simulink model "RELOrigin"  (R2022a)
settings: configuration reference "ChildModel" (kept outside this file)
libraries: simulink x4
(part 2 of 2)

== stateflow chart RELOrigin/REL/FRCenDoorRat ==
  state Initial
    en:
    SO_b_DoorRatRelaseReq=0;
    SO_DLKUnlockReq=0;
  state TRIGGER
    state DOOR_LOCK
      state REQ_UNLOCK
        en:
        SO_DLKUnlockReq=1;
      state SUCESS_UNLOCK
      state FAIL_UNLOCK
      (default) -> REQ_UNLOCK
      REQ_UNLOCK -> SUCESS_UNLOCK [order 1] : [SI_e_DoorLockSts==1]
      REQ_UNLOCK -> FAIL_UNLOCK [order 2] : [after(100,tick)&&...
          | SI_e_DoorLockSts==0]
    state RELEASE
      en:
      SO_b_DoorRatRelaseReq=1;
    state DOOR_UNLOCK
    (default) -> DOOR_LOCK [order 1] : [SI_e_DoorLockSts==0]
    DOOR_LOCK -> RELEASE : [SI_e_DoorLockSts==1&&...
        | SI_e_DoorRatSts!=3]
    DOOR_UNLOCK -> RELEASE : [SI_e_DoorLockSts==1&&...
        | SI_e_DoorRatSts!=3]
    (default) -> DOOR_UNLOCK [order 2]
  (default) -> Initial
  Initial -> TRIGGER : [!SI_b_OFF&&...
      | SI_e_DoorRatSts!=3&&...
      | ((SI_e_EspVehSpd<=0&&SI_b_EspVehSpdVld==0)||...
      | SI_e_VcuGearPosn==1)&&...
      | (hasChangedTo(SI_b_CdcDoorButtonSts,1)||...
      | hasChangedTo(SI_b_Cdc4DoorOpenButtonSts,1))]
  TRIGGER -> Initial : [hasChangedFrom(SI_e_VcuGearPosn,1)||...
      | (SI_e_EspVehSpd>=5&&SI_b_EspVehSpdVld==0)||...
      | (after(105,tick)&&SI_e_DoorLockSts==0)]
  RELEASE -> (junction 82) : [after(5,tick)]
  (junction 82) -> Initial
  data: SI_b_OFF input boolean; SO_b_DoorRatRelaseReq output boolean; SI_e_DoorLockSts input uint8; SI_e_EspVehSpd input uint8; SI_b_EspVehSpdVld input boolean; SI_e_DoorRatSts input uint8; SO_DLKUnlockReq output boolean; SI_e_VcuGearPosn input uint8; SI_b_CdcDoorButtonSts input boolean; SI_b_Cdc4DoorOpenButtonSts input boolean

== stateflow chart RELOrigin/REL/RLElecDoorRat ==
  state Initial
    en:
    SO_b_DoorRatRelaseReq=0;
  state RELEASE
    en:
    SO_b_DoorRatRelaseReq=1;
  (default) -> Initial
  Initial -> RELEASE : [!SI_b_OFF&&...
      | SI_e_DoorLockSts==1&&...
      | SI_e_DoorRatSts!=3&&...
      | ((SI_e_EspVehSpd<=0&&SI_b_EspVehSpdVld==0)||...
      | SI_e_VcuGearPosn==1)&&...
      | ((SI_e_BDCDoorHndSts==1&&hasChangedTo(SI_b_DoorHandleSW,1))||...
      | (SI_e_VcuGearPosn==1&&hasChangedTo(SI_e_BTDoorOpenReq,5))||...
      | (SI_e_VcuGearPosn==1&&hasChangedTo(SI_e_BTDoorOpenReq,9)))]
  RELEASE -> Initial : [after(5,tick)]
  data: SI_b_OFF input boolean; SO_b_DoorRatRelaseReq output boolean; SI_e_DoorLockSts input uint8; SI_e_EspVehSpd input uint8; SI_b_EspVehSpdVld input boolean; SI_e_DoorRatSts input uint8; SI_e_VcuGearPosn input uint8; SI_e_BDCDoorHndSts input uint8; SI_b_DoorHandleSW input boolean; SI_e_BTDoorOpenReq input uint8

== stateflow chart RELOrigin/REL/RLCenDoorRat ==
  state Initial
    en:
    SO_b_DoorRatRelaseReq=0;
    SO_DLKUnlockReq=0;
  state TRIGGER
    state DOOR_LOCK
      state REQ_UNLOCK
        en:
        SO_DLKUnlockReq=1;
      state SUCESS_UNLOCK
      state FAIL_UNLOCK
      (default) -> REQ_UNLOCK
      REQ_UNLOCK -> SUCESS_UNLOCK [order 1] : [SI_e_DoorLockSts==1]
      REQ_UNLOCK -> FAIL_UNLOCK [order 2] : [after(100,tick)&&...
          | SI_e_DoorLockSts==0]
    state RELEASE
      en:
      SO_b_DoorRatRelaseReq=1;
    state DOOR_UNLOCK
    (default) -> DOOR_LOCK [order 1] : [SI_e_DoorLockSts==0]
    DOOR_LOCK -> RELEASE : [SI_e_DoorLockSts==1&&...
        | SI_e_DoorRatSts!=3]
    DOOR_UNLOCK -> RELEASE : [SI_e_DoorLockSts==1&&...
        | SI_e_DoorRatSts!=3]
    (default) -> DOOR_UNLOCK [order 2]
  (default) -> Initial
  Initial -> TRIGGER : [!SI_b_OFF&&...
      | SI_e_DoorRatSts!=3&&...
      | ((SI_e_EspVehSpd<=0&&SI_b_EspVehSpdVld==0)||...
      | SI_e_VcuGearPosn==1)&&...
      | (hasChangedTo(SI_b_CdcDoorButtonSts,1)||...
      | hasChangedTo(SI_b_Cdc4DoorOpenButtonSts,1))]
  TRIGGER -> Initial : [hasChangedFrom(SI_e_VcuGearPosn,1)||...
      | (SI_e_EspVehSpd>=5&&SI_b_EspVehSpdVld==0)||...
      | (after(105,tick)&&SI_e_DoorLockSts==0)]
  RELEASE -> (junction 82) : [after(5,tick)]
  (junction 82) -> Initial
  data: SI_b_OFF input boolean; SO_b_DoorRatRelaseReq output boolean; SI_e_DoorLockSts input uint8; SI_e_EspVehSpd input uint8; SI_b_EspVehSpdVld input boolean; SI_e_DoorRatSts input uint8; SO_DLKUnlockReq output boolean; SI_e_VcuGearPosn input uint8; SI_b_CdcDoorButtonSts input boolean; SI_b_Cdc4DoorOpenButtonSts input boolean

== stateflow chart RELOrigin/REL/RRElecDoorRat ==
  state Initial
    en:
    SO_b_DoorRatRelaseReq=0;
  state RELEASE
    en:
    SO_b_DoorRatRelaseReq=1;
  (default) -> Initial
  Initial -> RELEASE : [!SI_b_OFF&&...
      | SI_e_DoorLockSts==1&&...
      | SI_e_DoorRatSts!=3&&...
      | ((SI_e_EspVehSpd<=0&&SI_b_EspVehSpdVld==0)||...
      | SI_e_VcuGearPosn==1)&&...
      | ((SI_e_BDCDoorHndSts==1&&hasChangedTo(SI_b_DoorHandleSW,1))||...
      | (SI_e_VcuGearPosn==1&&hasChangedTo(SI_e_BTDoorOpenReq,7))||...
      | (SI_e_VcuGearPosn==1&&hasChangedTo(SI_e_BTDoorOpenReq,9)))]
  RELEASE -> Initial : [after(5,tick)]
  data: SI_b_OFF input boolean; SO_b_DoorRatRelaseReq output boolean; SI_e_DoorLockSts input uint8; SI_e_EspVehSpd input uint8; SI_b_EspVehSpdVld input boolean; SI_e_DoorRatSts input uint8; SI_e_VcuGearPosn input uint8; SI_e_BDCDoorHndSts input uint8; SI_b_DoorHandleSW input boolean; SI_e_BTDoorOpenReq input uint8

== stateflow chart RELOrigin/REL/RRCenDoorRat ==
  state Initial
    en:
    SO_b_DoorRatRelaseReq=0;
    SO_DLKUnlockReq=0;
  state TRIGGER
    state DOOR_LOCK
      state REQ_UNLOCK
        en:
        SO_DLKUnlockReq=1;
      state SUCESS_UNLOCK
      state FAIL_UNLOCK
      (default) -> REQ_UNLOCK
      REQ_UNLOCK -> SUCESS_UNLOCK [order 1] : [SI_e_DoorLockSts==1]
      REQ_UNLOCK -> FAIL_UNLOCK [order 2] : [after(100,tick)&&...
          | SI_e_DoorLockSts==0]
    state RELEASE
      en:
      SO_b_DoorRatRelaseReq=1;
    state DOOR_UNLOCK
    (default) -> DOOR_LOCK [order 1] : [SI_e_DoorLockSts==0]
    DOOR_LOCK -> RELEASE : [SI_e_DoorLockSts==1&&...
        | SI_e_DoorRatSts!=3]
    DOOR_UNLOCK -> RELEASE : [SI_e_DoorLockSts==1&&...
        | SI_e_DoorRatSts!=3]
    (default) -> DOOR_UNLOCK [order 2]
  (default) -> Initial
  Initial -> TRIGGER : [!SI_b_OFF&&...
      | SI_e_DoorRatSts!=3&&...
      | ((SI_e_EspVehSpd<=0&&SI_b_EspVehSpdVld==0)||...
      | SI_e_VcuGearPosn==1)&&...
      | (hasChangedTo(SI_b_CdcDoorButtonSts,1)||...
      | hasChangedTo(SI_b_Cdc4DoorOpenButtonSts,1))]
  TRIGGER -> Initial : [hasChangedFrom(SI_e_VcuGearPosn,1)||...
      | (SI_e_EspVehSpd>=5&&SI_b_EspVehSpdVld==0)||...
      | (after(105,tick)&&SI_e_DoorLockSts==0)]
  RELEASE -> (junction 82) : [after(5,tick)]
  (junction 82) -> Initial
  data: SI_b_OFF input boolean; SO_b_DoorRatRelaseReq output boolean; SI_e_DoorLockSts input uint8; SI_e_EspVehSpd input uint8; SI_b_EspVehSpdVld input boolean; SI_e_DoorRatSts input uint8; SO_DLKUnlockReq output boolean; SI_e_VcuGearPosn input uint8; SI_b_CdcDoorButtonSts input boolean; SI_b_Cdc4DoorOpenButtonSts input boolean

== stateflow chart RELOrigin/REL/FLDoorReleaseDriver ==
  state STARTUP_SETTING
    en:
    SO_b_MotorA=0;
    SO_b_MotorB=1;
    SO_e_MotorMode=2;
  state NORMAL
    state ELECTRIC_DOOR
      state MAIN_PROGRESS [parallel]
        settings: executionOrder=1
        state RELEASE
          en:
          SL_e_CheckCycle=0;
          state STEP2_OPEN
            state IDLE
              en:
              SO_b_MotorA=0;
              SO_b_MotorB=0;
              SO_e_MotorMode=0;
            state WAITING
            state ERROR
              en:
              SO_b_Error=1;
            state LAST_CHECK
            state ICE_BREAK
            state ERROR1
              en:
              SO_b_Error=1;
            (default) -> NORMAL.ELECTRIC_DOOR.MAIN_PROGRESS.RELEASE.STEP2_OPEN.IDLE
            NORMAL.ELECTRIC_DOOR.MAIN_PROGRESS.RELEASE.STEP2_OPEN.IDLE -> NORMAL.ELECTRIC_DOOR.MAIN_PROGRESS.RELEASE.STEP2_OPEN.WAITING [order 1] : [SI_b_DoorOpenSts==1]
            NORMAL.ELECTRIC_DOOR.MAIN_PROGRESS.RELEASE.STEP2_OPEN.WAITING -> (junction 227) : [after(5,tick)]
            (junction 227) -> (junction 226)
            NORMAL.ELECTRIC_DOOR.MAIN_PROGRESS.RELEASE.STEP2_OPEN.IDLE -> (junction 226) [order 2] : [before(270,tick)&&...
                | hasChangedTo(SI_b_DoorOpenSts,1)]
            (junction 226) -> (junction 219)
            NORMAL.ELECTRIC_DOOR.MAIN_PROGRESS.RELEASE.STEP2_OPEN.IDLE -> NORMAL.ELECTRIC_DOOR.MAIN_PROGRESS.RELEASE.STEP2_OPEN.LAST_CHECK [order 3] : [after(300,tick)&&...
                | SI_b_DoorOpenSts==0]
            ERROR -> (junction 219) : [after(5,tick)]
            NORMAL.ELECTRIC_DOOR.MAIN_PROGRESS.RELEASE.STEP2_OPEN.LAST_CHECK -> ERROR [order 1] : [SI_b_DCUCinchHomeSwt!=1]
            (junction 219) -> (junction 210)
            NORMAL.ELECTRIC_DOOR.MAIN_PROGRESS.RELEASE.STEP2_OPEN.LAST_CHECK -> ICE_BREAK [order 2] : [SI_b_DCUCinchHomeSwt==1]
            ICE_BREAK -> ERROR1 [order 2] : [after(600,tick)&&...
                | SI_b_DCUCinchHomeSwt==1]
            ERROR1 -> (junction 210) : [after(5,tick)]
            (junction 210) -> (junction 225)
            ICE_BREAK -> (junction 225) [order 1] : [before(600,tick)&&...
                | hasChangedTo(SI_b_DCUCinchHomeSwt,0)]
          state INITIAL
            en:
            SO_b_MotorA=1;
            SO_b_MotorB=0;
            SO_e_MotorMode=1;
            //MotorA=Release Side
          state CHECKING
            en:
            SO_b_MotorA=0;
            SO_b_MotorB=0;
            SO_e_MotorMode=0;
            SL_e_CheckCycle++;
          state RESET
            en:
            SO_b_MotorA=0;
            SO_b_MotorB=1;
            SO_e_MotorMode=2;
          (default) -> NORMAL.ELECTRIC_DOOR.MAIN_PROGRESS.RELEASE.INITIAL
          NORMAL.ELECTRIC_DOOR.MAIN_PROGRESS.RELEASE.INITIAL -> NORMAL.ELECTRIC_DOOR.MAIN_PROGRESS.RELEASE.CHECKING : [after(30,tick)]
          NORMAL.ELECTRIC_DOOR.MAIN_PROGRESS.RELEASE.CHECKING -> NORMAL.ELECTRIC_DOOR.MAIN_PROGRESS.RELEASE.INITIAL [order 2] : [after(5,tick)&&...
              | SI_b_DoorAjarSts!=1&&...
              | SL_e_CheckCycle<2]
          NORMAL.ELECTRIC_DOOR.MAIN_PROGRESS.RELEASE.CHECKING -> NORMAL.ELECTRIC_DOOR.MAIN_PROGRESS.RELEASE.STEP2_OPEN [order 1] : [after(5,tick)&&...
              | SI_b_DoorAjarSts==1]
          NORMAL.ELECTRIC_DOOR.MAIN_PROGRESS.RELEASE.CHECKING -> NORMAL.ELECTRIC_DOOR.MAIN_PROGRESS.RELEASE.RESET [order 3] : [after(5,tick)&&...
              | SI_b_DoorAjarSts!=1&&...
              | SL_e_CheckCycle>=2]
          (junction 225) -> NORMAL.ELECTRIC_DOOR.MAIN_PROGRESS.RELEASE.RESET
        state IDLE
          en:
          SO_b_MotorA=0;
          SO_b_MotorB=0;
          SO_e_MotorMode=0;
          SO_b_Error=0;
        (default) -> NORMAL.ELECTRIC_DOOR.MAIN_PROGRESS.IDLE
        NORMAL.ELECTRIC_DOOR.MAIN_PROGRESS.IDLE -> NORMAL.ELECTRIC_DOOR.MAIN_PROGRESS.RELEASE : [hasChangedTO(SI_b_TriggerRelease,1)]
        NORMAL.ELECTRIC_DOOR.MAIN_PROGRESS.RELEASE.RESET -> NORMAL.ELECTRIC_DOOR.MAIN_PROGRESS.IDLE : [after(30,tick)]
    state NON_ELECTRIC_DOOR
      state MAIN_PROGRESS [parallel]
        settings: executionOrder=1
        state RELEASE
          en:
          SL_e_CheckCycle=0;
          state INITIAL
            en:
            SO_b_MotorA=1;
            SO_b_MotorB=0;
            SO_e_MotorMode=1;
            //MotorA=Release Side
          state CHECKING
            en:
            SO_b_MotorA=0;
            SO_b_MotorB=0;
            SO_e_MotorMode=0;
            SL_e_CheckCycle++;
          state STEP2_OPEN
            state IDLE
              en:
              SO_b_MotorA=0;
              SO_b_MotorB=0;
              SO_e_MotorMode=0;
            state WAITING
            state LAST_CHECK
            (default) -> NORMAL.NON_ELECTRIC_DOOR.MAIN_PROGRESS.RELEASE.STEP2_OPEN.IDLE
            NORMAL.NON_ELECTRIC_DOOR.MAIN_PROGRESS.RELEASE.STEP2_OPEN.WAITING -> (junction 251) : [after(5,tick)]
            NORMAL.NON_ELECTRIC_DOOR.MAIN_PROGRESS.RELEASE.STEP2_OPEN.IDLE -> NORMAL.NON_ELECTRIC_DOOR.MAIN_PROGRESS.RELEASE.STEP2_OPEN.WAITING [order 1] : [SI_b_DoorOpenSts==1]
            (junction 251) -> (junction 250)
            NORMAL.NON_ELECTRIC_DOOR.MAIN_PROGRESS.RELEASE.STEP2_OPEN.IDLE -> (junction 250) [order 2] : [before(270,tick)&&...
                | hasChangedTo(SI_b_DoorOpenSts,1)]
            (junction 250) -> (junction 242)
            NORMAL.NON_ELECTRIC_DOOR.MAIN_PROGRESS.RELEASE.STEP2_OPEN.IDLE -> NORMAL.NON_ELECTRIC_DOOR.MAIN_PROGRESS.RELEASE.STEP2_OPEN.LAST_CHECK [order 3] : [after(300,tick)&&...
                | SI_b_DoorOpenSts==0]
            NORMAL.NON_ELECTRIC_DOOR.MAIN_PROGRESS.RELEASE.STEP2_OPEN.LAST_CHECK -> (junction 242)
          state RESET
            en:
            SO_b_MotorA=0;
            SO_b_MotorB=1;
            SO_e_MotorMode=2;
          (default) -> NORMAL.NON_ELECTRIC_DOOR.MAIN_PROGRESS.RELEASE.INITIAL
          NORMAL.NON_ELECTRIC_DOOR.MAIN_PROGRESS.RELEASE.INITIAL -> NORMAL.NON_ELECTRIC_DOOR.MAIN_PROGRESS.RELEASE.CHECKING : [after(30,tick)]
          NORMAL.NON_ELECTRIC_DOOR.MAIN_PROGRESS.RELEASE.CHECKING -> NORMAL.NON_ELECTRIC_DOOR.MAIN_PROGRESS.RELEASE.STEP2_OPEN [order 1] : [after(5,tick)&&...
              | SI_b_DoorAjarSts==1]
          NORMAL.NON_ELECTRIC_DOOR.MAIN_PROGRESS.RELEASE.CHECKING -> NORMAL.NON_ELECTRIC_DOOR.MAIN_PROGRESS.RELEASE.INITIAL [order 2] : [after(5,tick)&&...
              | SI_b_DoorAjarSts!=1&&...
              | SL_e_CheckCycle<2]
          NORMAL.NON_ELECTRIC_DOOR.MAIN_PROGRESS.RELEASE.CHECKING -> NORMAL.NON_ELECTRIC_DOOR.MAIN_PROGRESS.RELEASE.RESET [order 3] : [after(5,tick)&&...
              | SI_b_DoorAjarSts!=1&&...
              | SL_e_CheckCycle>=2]
          (junction 242) -> NORMAL.NON_ELECTRIC_DOOR.MAIN_PROGRESS.RELEASE.RESET
        state IDLE
          en:
          SO_b_MotorA=0;
          SO_b_MotorB=0;
          SO_e_MotorMode=0;
        (default) -> NORMAL.NON_ELECTRIC_DOOR.MAIN_PROGRESS.IDLE
        NORMAL.NON_ELECTRIC_DOOR.MAIN_PROGRESS.IDLE -> NORMAL.NON_ELECTRIC_DOOR.MAIN_PROGRESS.RELEASE : [hasChangedTO(SI_b_TriggerRelease,1)]
        NORMAL.NON_ELECTRIC_DOOR.MAIN_PROGRESS.RELEASE.RESET -> NORMAL.NON_ELECTRIC_DOOR.MAIN_PROGRESS.IDLE : [after(30,tick)]
    (default) -> ELECTRIC_DOOR [order 1] : [SI_b_ElectricDoorCfg]
    (default) -> NON_ELECTRIC_DOOR [order 2]
  (default) -> STARTUP_SETTING
  STARTUP_SETTING -> NORMAL : [after(30,tick)]
  data: SO_b_MotorA output boolean; SI_b_TriggerRelease input boolean; SI_b_DoorOpenSts input boolean; SO_b_MotorB output boolean; SO_e_MotorMode output uint8; SI_b_DCUCinchHomeSwt input boolean; SO_b_Error output boolean; SI_b_ElectricDoorCfg input boolean; SI_b_DoorAjarSts input boolean

== stateflow chart RELOrigin/REL/FRDoorReleaseDriver ==
  state STARTUP_SETTING
    en:
    SO_b_MotorA=0;
    SO_b_MotorB=1;
    SO_e_MotorMode=2;
  state NORMAL
    state ELECTRIC_DOOR
      state MAIN_PROGRESS [parallel]
        settings: executionOrder=1
        state RELEASE
          en:
          SL_e_CheckCycle=0;
          state STEP2_OPEN
            state IDLE
              en:
              SO_b_MotorA=0;
              SO_b_MotorB=0;
              SO_e_MotorMode=0;
            state WAITING
            state ERROR
              en:
              SO_b_Error=1;
            state LAST_CHECK
            state ICE_BREAK
            state ERROR1
              en:
              SO_b_Error=1;
            (default) -> NORMAL.ELECTRIC_DOOR.MAIN_PROGRESS.RELEASE.STEP2_OPEN.IDLE
            NORMAL.ELECTRIC_DOOR.MAIN_PROGRESS.RELEASE.STEP2_OPEN.IDLE -> NORMAL.ELECTRIC_DOOR.MAIN_PROGRESS.RELEASE.STEP2_OPEN.WAITING [order 1] : [SI_b_DoorOpenSts==1]
            NORMAL.ELECTRIC_DOOR.MAIN_PROGRESS.RELEASE.STEP2_OPEN.WAITING -> (junction 227) : [after(5,tick)]
            (junction 227) -> (junction 226)
            NORMAL.ELECTRIC_DOOR.MAIN_PROGRESS.RELEASE.STEP2_OPEN.IDLE -> (junction 226) [order 2] : [before(270,tick)&&...
                | hasChangedTo(SI_b_DoorOpenSts,1)]
            (junction 226) -> (junction 219)
            NORMAL.ELECTRIC_DOOR.MAIN_PROGRESS.RELEASE.STEP2_OPEN.IDLE -> NORMAL.ELECTRIC_DOOR.MAIN_PROGRESS.RELEASE.STEP2_OPEN.LAST_CHECK [order 3] : [after(300,tick)&&...
                | SI_b_DoorOpenSts==0]
            ERROR -> (junction 219) : [after(5,tick)]
            NORMAL.ELECTRIC_DOOR.MAIN_PROGRESS.RELEASE.STEP2_OPEN.LAST_CHECK -> ERROR [order 1] : [SI_b_DCUCinchHomeSwt!=1]
            (junction 219) -> (junction 210)
            NORMAL.ELECTRIC_DOOR.MAIN_PROGRESS.RELEASE.STEP2_OPEN.LAST_CHECK -> ICE_BREAK [order 2] : [SI_b_DCUCinchHomeSwt==1]
            ICE_BREAK -> ERROR1 [order 2] : [after(600,tick)&&...
                | SI_b_DCUCinchHomeSwt==1]
            ERROR1 -> (junction 210) : [after(5,tick)]
            (junction 210) -> (junction 225)
            ICE_BREAK -> (junction 225) [order 1] : [before(600,tick)&&...
                | hasChangedTo(SI_b_DCUCinchHomeSwt,0)]
          state INITIAL
            en:
            SO_b_MotorA=1;
            SO_b_MotorB=0;
            SO_e_MotorMode=1;
            //MotorA=Release Side
          state CHECKING
            en:
            SO_b_MotorA=0;
            SO_b_MotorB=0;
            SO_e_MotorMode=0;
            SL_e_CheckCycle++;
          state RESET
            en:
            SO_b_MotorA=0;
            SO_b_MotorB=1;
            SO_e_MotorMode=2;
          (default) -> NORMAL.ELECTRIC_DOOR.MAIN_PROGRESS.RELEASE.INITIAL
          NORMAL.ELECTRIC_DOOR.MAIN_PROGRESS.RELEASE.INITIAL -> NORMAL.ELECTRIC_DOOR.MAIN_PROGRESS.RELEASE.CHECKING : [after(30,tick)]
          NORMAL.ELECTRIC_DOOR.MAIN_PROGRESS.RELEASE.CHECKING -> NORMAL.ELECTRIC_DOOR.MAIN_PROGRESS.RELEASE.INITIAL [order 2] : [after(5,tick)&&...
              | SI_b_DoorAjarSts!=1&&...
              | SL_e_CheckCycle<2]
          NORMAL.ELECTRIC_DOOR.MAIN_PROGRESS.RELEASE.CHECKING -> NORMAL.ELECTRIC_DOOR.MAIN_PROGRESS.RELEASE.STEP2_OPEN [order 1] : [after(5,tick)&&...
              | SI_b_DoorAjarSts==1]
          NORMAL.ELECTRIC_DOOR.MAIN_PROGRESS.RELEASE.CHECKING -> NORMAL.ELECTRIC_DOOR.MAIN_PROGRESS.RELEASE.RESET [order 3] : [after(5,tick)&&...
              | SI_b_DoorAjarSts!=1&&...
              | SL_e_CheckCycle>=2]
          (junction 225) -> NORMAL.ELECTRIC_DOOR.MAIN_PROGRESS.RELEASE.RESET
        state IDLE
          en:
          SO_b_MotorA=0;
          SO_b_MotorB=0;
          SO_e_MotorMode=0;
          SO_b_Error=0;
        (default) -> NORMAL.ELECTRIC_DOOR.MAIN_PROGRESS.IDLE
        NORMAL.ELECTRIC_DOOR.MAIN_PROGRESS.IDLE -> NORMAL.ELECTRIC_DOOR.MAIN_PROGRESS.RELEASE : [hasChangedTO(SI_b_TriggerRelease,1)]
        NORMAL.ELECTRIC_DOOR.MAIN_PROGRESS.RELEASE.RESET -> NORMAL.ELECTRIC_DOOR.MAIN_PROGRESS.IDLE : [after(30,tick)]
    state NON_ELECTRIC_DOOR
      state MAIN_PROGRESS [parallel]
        settings: executionOrder=1
        state RELEASE
          en:
          SL_e_CheckCycle=0;
          state INITIAL
            en:
            SO_b_MotorA=1;
            SO_b_MotorB=0;
            SO_e_MotorMode=1;
            //MotorA=Release Side
          state CHECKING
            en:
            SO_b_MotorA=0;
            SO_b_MotorB=0;
            SO_e_MotorMode=0;
            SL_e_CheckCycle++;
          state STEP2_OPEN
            state IDLE
              en:
              SO_b_MotorA=0;
              SO_b_MotorB=0;
              SO_e_MotorMode=0;
            state WAITING
            state LAST_CHECK
            (default) -> NORMAL.NON_ELECTRIC_DOOR.MAIN_PROGRESS.RELEASE.STEP2_OPEN.IDLE
            NORMAL.NON_ELECTRIC_DOOR.MAIN_PROGRESS.RELEASE.STEP2_OPEN.WAITING -> (junction 251) : [after(5,tick)]
            NORMAL.NON_ELECTRIC_DOOR.MAIN_PROGRESS.RELEASE.STEP2_OPEN.IDLE -> NORMAL.NON_ELECTRIC_DOOR.MAIN_PROGRESS.RELEASE.STEP2_OPEN.WAITING [order 1] : [SI_b_DoorOpenSts==1]
            (junction 251) -> (junction 250)
            NORMAL.NON_ELECTRIC_DOOR.MAIN_PROGRESS.RELEASE.STEP2_OPEN.IDLE -> (junction 250) [order 2] : [before(270,tick)&&...
                | hasChangedTo(SI_b_DoorOpenSts,1)]
            (junction 250) -> (junction 242)
            NORMAL.NON_ELECTRIC_DOOR.MAIN_PROGRESS.RELEASE.STEP2_OPEN.IDLE -> NORMAL.NON_ELECTRIC_DOOR.MAIN_PROGRESS.RELEASE.STEP2_OPEN.LAST_CHECK [order 3] : [after(300,tick)&&...
                | SI_b_DoorOpenSts==0]
            NORMAL.NON_ELECTRIC_DOOR.MAIN_PROGRESS.RELEASE.STEP2_OPEN.LAST_CHECK -> (junction 242)
          state RESET
            en:
            SO_b_MotorA=0;
            SO_b_MotorB=1;
            SO_e_MotorMode=2;
          (default) -> NORMAL.NON_ELECTRIC_DOOR.MAIN_PROGRESS.RELEASE.INITIAL
          NORMAL.NON_ELECTRIC_DOOR.MAIN_PROGRESS.RELEASE.INITIAL -> NORMAL.NON_ELECTRIC_DOOR.MAIN_PROGRESS.RELEASE.CHECKING : [after(30,tick)]
          NORMAL.NON_ELECTRIC_DOOR.MAIN_PROGRESS.RELEASE.CHECKING -> NORMAL.NON_ELECTRIC_DOOR.MAIN_PROGRESS.RELEASE.STEP2_OPEN [order 1] : [after(5,tick)&&...
              | SI_b_DoorAjarSts==1]
          NORMAL.NON_ELECTRIC_DOOR.MAIN_PROGRESS.RELEASE.CHECKING -> NORMAL.NON_ELECTRIC_DOOR.MAIN_PROGRESS.RELEASE.INITIAL [order 2] : [after(5,tick)&&...
              | SI_b_DoorAjarSts!=1&&...
              | SL_e_CheckCycle<2]
          NORMAL.NON_ELECTRIC_DOOR.MAIN_PROGRESS.RELEASE.CHECKING -> NORMAL.NON_ELECTRIC_DOOR.MAIN_PROGRESS.RELEASE.RESET [order 3] : [after(5,tick)&&...
              | SI_b_DoorAjarSts!=1&&...
              | SL_e_CheckCycle>=2]
          (junction 242) -> NORMAL.NON_ELECTRIC_DOOR.MAIN_PROGRESS.RELEASE.RESET
        state IDLE
          en:
          SO_b_MotorA=0;
          SO_b_MotorB=0;
          SO_e_MotorMode=0;
        (default) -> NORMAL.NON_ELECTRIC_DOOR.MAIN_PROGRESS.IDLE
        NORMAL.NON_ELECTRIC_DOOR.MAIN_PROGRESS.IDLE -> NORMAL.NON_ELECTRIC_DOOR.MAIN_PROGRESS.RELEASE : [hasChangedTO(SI_b_TriggerRelease,1)]
        NORMAL.NON_ELECTRIC_DOOR.MAIN_PROGRESS.RELEASE.RESET -> NORMAL.NON_ELECTRIC_DOOR.MAIN_PROGRESS.IDLE : [after(30,tick)]
    (default) -> ELECTRIC_DOOR [order 1] : [SI_b_ElectricDoorCfg]
    (default) -> NON_ELECTRIC_DOOR [order 2]
  (default) -> STARTUP_SETTING
  STARTUP_SETTING -> NORMAL : [after(30,tick)]
  data: SO_b_MotorA output boolean; SI_b_TriggerRelease input boolean; SI_b_DoorOpenSts input boolean; SO_b_MotorB output boolean; SO_e_MotorMode output uint8; SI_b_DCUCinchHomeSwt input boolean; SO_b_Error output boolean; SI_b_ElectricDoorCfg input boolean; SI_b_DoorAjarSts input boolean

== stateflow chart RELOrigin/REL/RLDoorReleaseDriver ==
  state STARTUP_SETTING
    en:
    SO_b_MotorA=0;
    SO_b_MotorB=1;
    SO_e_MotorMode=2;
  state NORMAL
    state ELECTRIC_DOOR
      state MAIN_PROGRESS [parallel]
        settings: executionOrder=1
        state RELEASE
          en:
          SL_e_CheckCycle=0;
          state STEP2_OPEN
            state IDLE
              en:
              SO_b_MotorA=0;
              SO_b_MotorB=0;
              SO_e_MotorMode=0;
            state WAITING
            state ERROR
              en:
              SO_b_Error=1;
            state LAST_CHECK
            state ICE_BREAK
            state ERROR1
              en:
              SO_b_Error=1;
            (default) -> NORMAL.ELECTRIC_DOOR.MAIN_PROGRESS.RELEASE.STEP2_OPEN.IDLE
            NORMAL.ELECTRIC_DOOR.MAIN_PROGRESS.RELEASE.STEP2_OPEN.IDLE -> NORMAL.ELECTRIC_DOOR.MAIN_PROGRESS.RELEASE.STEP2_OPEN.WAITING [order 1] : [SI_b_DoorOpenSts==1]
            NORMAL.ELECTRIC_DOOR.MAIN_PROGRESS.RELEASE.STEP2_OPEN.WAITING -> (junction 227) : [after(5,tick)]
            (junction 227) -> (junction 226)
            NORMAL.ELECTRIC_DOOR.MAIN_PROGRESS.RELEASE.STEP2_OPEN.IDLE -> (junction 226) [order 2] : [before(270,tick)&&...
                | hasChangedTo(SI_b_DoorOpenSts,1)]
            (junction 226) -> (junction 219)
            NORMAL.ELECTRIC_DOOR.MAIN_PROGRESS.RELEASE.STEP2_OPEN.IDLE -> NORMAL.ELECTRIC_DOOR.MAIN_PROGRESS.RELEASE.STEP2_OPEN.LAST_CHECK [order 3] : [after(300,tick)&&...
                | SI_b_DoorOpenSts==0]
            ERROR -> (junction 219) : [after(5,tick)]
            NORMAL.ELECTRIC_DOOR.MAIN_PROGRESS.RELEASE.STEP2_OPEN.LAST_CHECK -> ERROR [order 1] : [SI_b_DCUCinchHomeSwt!=1]
            (junction 219) -> (junction 210)
            NORMAL.ELECTRIC_DOOR.MAIN_PROGRESS.RELEASE.STEP2_OPEN.LAST_CHECK -> ICE_BREAK [order 2] : [SI_b_DCUCinchHomeSwt==1]
            ICE_BREAK -> ERROR1 [order 2] : [after(600,tick)&&...
                | SI_b_DCUCinchHomeSwt==1]
            ERROR1 -> (junction 210) : [after(5,tick)]
            (junction 210) -> (junction 225)
            ICE_BREAK -> (junction 225) [order 1] : [before(600,tick)&&...
                | hasChangedTo(SI_b_DCUCinchHomeSwt,0)]
          state INITIAL
            en:
            SO_b_MotorA=1;
            SO_b_MotorB=0;
            SO_e_MotorMode=1;
            //MotorA=Release Side
          state CHECKING
            en:
            SO_b_MotorA=0;
            SO_b_MotorB=0;
            SO_e_MotorMode=0;
            SL_e_CheckCycle++;
          state RESET
            en:
            SO_b_MotorA=0;
            SO_b_MotorB=1;
            SO_e_MotorMode=2;
          (default) -> NORMAL.ELECTRIC_DOOR.MAIN_PROGRESS.RELEASE.INITIAL
          NORMAL.ELECTRIC_DOOR.MAIN_PROGRESS.RELEASE.INITIAL -> NORMAL.ELECTRIC_DOOR.MAIN_PROGRESS.RELEASE.CHECKING : [after(30,tick)]
          NORMAL.ELECTRIC_DOOR.MAIN_PROGRESS.RELEASE.CHECKING -> NORMAL.ELECTRIC_DOOR.MAIN_PROGRESS.RELEASE.INITIAL [order 2] : [after(5,tick)&&...
              | SI_b_DoorAjarSts!=1&&...
              | SL_e_CheckCycle<2]
          NORMAL.ELECTRIC_DOOR.MAIN_PROGRESS.RELEASE.CHECKING -> NORMAL.ELECTRIC_DOOR.MAIN_PROGRESS.RELEASE.STEP2_OPEN [order 1] : [after(5,tick)&&...
              | SI_b_DoorAjarSts==1]
          NORMAL.ELECTRIC_DOOR.MAIN_PROGRESS.RELEASE.CHECKING -> NORMAL.ELECTRIC_DOOR.MAIN_PROGRESS.RELEASE.RESET [order 3] : [after(5,tick)&&...
              | SI_b_DoorAjarSts!=1&&...
              | SL_e_CheckCycle>=2]
          (junction 225) -> NORMAL.ELECTRIC_DOOR.MAIN_PROGRESS.RELEASE.RESET
        state IDLE
          en:
          SO_b_MotorA=0;
          SO_b_MotorB=0;
          SO_e_MotorMode=0;
          SO_b_Error=0;
        (default) -> NORMAL.ELECTRIC_DOOR.MAIN_PROGRESS.IDLE
        NORMAL.ELECTRIC_DOOR.MAIN_PROGRESS.IDLE -> NORMAL.ELECTRIC_DOOR.MAIN_PROGRESS.RELEASE : [hasChangedTO(SI_b_TriggerRelease,1)]
        NORMAL.ELECTRIC_DOOR.MAIN_PROGRESS.RELEASE.RESET -> NORMAL.ELECTRIC_DOOR.MAIN_PROGRESS.IDLE : [after(30,tick)]
    state NON_ELECTRIC_DOOR
      state MAIN_PROGRESS [parallel]
        settings: executionOrder=1
        state RELEASE
          en:
          SL_e_CheckCycle=0;
          state INITIAL
            en:
            SO_b_MotorA=1;
            SO_b_MotorB=0;
            SO_e_MotorMode=1;
            //MotorA=Release Side
          state CHECKING
            en:
            SO_b_MotorA=0;
            SO_b_MotorB=0;
            SO_e_MotorMode=0;
            SL_e_CheckCycle++;
          state STEP2_OPEN
            state IDLE
              en:
              SO_b_MotorA=0;
              SO_b_MotorB=0;
              SO_e_MotorMode=0;
            state WAITING
            state LAST_CHECK
            (default) -> NORMAL.NON_ELECTRIC_DOOR.MAIN_PROGRESS.RELEASE.STEP2_OPEN.IDLE
            NORMAL.NON_ELECTRIC_DOOR.MAIN_PROGRESS.RELEASE.STEP2_OPEN.WAITING -> (junction 251) : [after(5,tick)]
            NORMAL.NON_ELECTRIC_DOOR.MAIN_PROGRESS.RELEASE.STEP2_OPEN.IDLE -> NORMAL.NON_ELECTRIC_DOOR.MAIN_PROGRESS.RELEASE.STEP2_OPEN.WAITING [order 1] : [SI_b_DoorOpenSts==1]
            (junction 251) -> (junction 250)
            NORMAL.NON_ELECTRIC_DOOR.MAIN_PROGRESS.RELEASE.STEP2_OPEN.IDLE -> (junction 250) [order 2] : [before(270,tick)&&...
                | hasChangedTo(SI_b_DoorOpenSts,1)]
            (junction 250) -> (junction 242)
            NORMAL.NON_ELECTRIC_DOOR.MAIN_PROGRESS.RELEASE.STEP2_OPEN.IDLE -> NORMAL.NON_ELECTRIC_DOOR.MAIN_PROGRESS.RELEASE.STEP2_OPEN.LAST_CHECK [order 3] : [after(300,tick)&&...
                | SI_b_DoorOpenSts==0]
            NORMAL.NON_ELECTRIC_DOOR.MAIN_PROGRESS.RELEASE.STEP2_OPEN.LAST_CHECK -> (junction 242)
          state RESET
            en:
            SO_b_MotorA=0;
            SO_b_MotorB=1;
            SO_e_MotorMode=2;
          (default) -> NORMAL.NON_ELECTRIC_DOOR.MAIN_PROGRESS.RELEASE.INITIAL
          NORMAL.NON_ELECTRIC_DOOR.MAIN_PROGRESS.RELEASE.INITIAL -> NORMAL.NON_ELECTRIC_DOOR.MAIN_PROGRESS.RELEASE.CHECKING : [after(30,tick)]
          NORMAL.NON_ELECTRIC_DOOR.MAIN_PROGRESS.RELEASE.CHECKING -> NORMAL.NON_ELECTRIC_DOOR.MAIN_PROGRESS.RELEASE.STEP2_OPEN [order 1] : [after(5,tick)&&...
              | SI_b_DoorAjarSts==1]
          NORMAL.NON_ELECTRIC_DOOR.MAIN_PROGRESS.RELEASE.CHECKING -> NORMAL.NON_ELECTRIC_DOOR.MAIN_PROGRESS.RELEASE.INITIAL [order 2] : [after(5,tick)&&...
              | SI_b_DoorAjarSts!=1&&...
              | SL_e_CheckCycle<2]
          NORMAL.NON_ELECTRIC_DOOR.MAIN_PROGRESS.RELEASE.CHECKING -> NORMAL.NON_ELECTRIC_DOOR.MAIN_PROGRESS.RELEASE.RESET [order 3] : [after(5,tick)&&...
              | SI_b_DoorAjarSts!=1&&...
              | SL_e_CheckCycle>=2]
          (junction 242) -> NORMAL.NON_ELECTRIC_DOOR.MAIN_PROGRESS.RELEASE.RESET
        state IDLE
          en:
          SO_b_MotorA=0;
          SO_b_MotorB=0;
          SO_e_MotorMode=0;
        (default) -> NORMAL.NON_ELECTRIC_DOOR.MAIN_PROGRESS.IDLE
        NORMAL.NON_ELECTRIC_DOOR.MAIN_PROGRESS.IDLE -> NORMAL.NON_ELECTRIC_DOOR.MAIN_PROGRESS.RELEASE : [hasChangedTO(SI_b_TriggerRelease,1)]
        NORMAL.NON_ELECTRIC_DOOR.MAIN_PROGRESS.RELEASE.RESET -> NORMAL.NON_ELECTRIC_DOOR.MAIN_PROGRESS.IDLE : [after(30,tick)]
    (default) -> ELECTRIC_DOOR [order 1] : [SI_b_ElectricDoorCfg]
    (default) -> NON_ELECTRIC_DOOR [order 2]
  (default) -> STARTUP_SETTING
  STARTUP_SETTING -> NORMAL : [after(30,tick)]
  data: SO_b_MotorA output boolean; SI_b_TriggerRelease input boolean; SI_b_DoorOpenSts input boolean; SO_b_MotorB output boolean; SO_e_MotorMode output uint8; SI_b_DCUCinchHomeSwt input boolean; SO_b_Error output boolean; SI_b_ElectricDoorCfg input boolean; SI_b_DoorAjarSts input boolean

== stateflow chart RELOrigin/REL/RLDoorReleaseDriver1 ==
  state STARTUP_SETTING
    en:
    SO_b_MotorA=0;
    SO_b_MotorB=1;
    SO_e_MotorMode=2;
  state NORMAL
    state ELECTRIC_DOOR
      state MAIN_PROGRESS [parallel]
        settings: executionOrder=1
        state RELEASE
          en:
          SL_e_CheckCycle=0;
          state STEP2_OPEN
            state IDLE
              en:
              SO_b_MotorA=0;
              SO_b_MotorB=0;
              SO_e_MotorMode=0;
            state WAITING
            state ERROR
              en:
              SO_b_Error=1;
            state LAST_CHECK
            state ICE_BREAK
            state ERROR1
              en:
              SO_b_Error=1;
            (default) -> NORMAL.ELECTRIC_DOOR.MAIN_PROGRESS.RELEASE.STEP2_OPEN.IDLE
            NORMAL.ELECTRIC_DOOR.MAIN_PROGRESS.RELEASE.STEP2_OPEN.IDLE -> NORMAL.ELECTRIC_DOOR.MAIN_PROGRESS.RELEASE.STEP2_OPEN.WAITING [order 1] : [SI_b_DoorOpenSts==1]
            NORMAL.ELECTRIC_DOOR.MAIN_PROGRESS.RELEASE.STEP2_OPEN.WAITING -> (junction 227) : [after(5,tick)]
            (junction 227) -> (junction 226)
            NORMAL.ELECTRIC_DOOR.MAIN_PROGRESS.RELEASE.STEP2_OPEN.IDLE -> (junction 226) [order 2] : [before(270,tick)&&...
                | hasChangedTo(SI_b_DoorOpenSts,1)]
            (junction 226) -> (junction 219)
            NORMAL.ELECTRIC_DOOR.MAIN_PROGRESS.RELEASE.STEP2_OPEN.IDLE -> NORMAL.ELECTRIC_DOOR.MAIN_PROGRESS.RELEASE.STEP2_OPEN.LAST_CHECK [order 3] : [after(300,tick)&&...
                | SI_b_DoorOpenSts==0]
            ERROR -> (junction 219) : [after(5,tick)]
            NORMAL.ELECTRIC_DOOR.MAIN_PROGRESS.RELEASE.STEP2_OPEN.LAST_CHECK -> ERROR [order 1] : [SI_b_DCUCinchHomeSwt!=1]
            (junction 219) -> (junction 210)
            NORMAL.ELECTRIC_DOOR.MAIN_PROGRESS.RELEASE.STEP2_OPEN.LAST_CHECK -> ICE_BREAK [order 2] : [SI_b_DCUCinchHomeSwt==1]
            ICE_BREAK -> ERROR1 [order 2] : [after(600,tick)&&...
                | SI_b_DCUCinchHomeSwt==1]
            ERROR1 -> (junction 210) : [after(5,tick)]
            (junction 210) -> (junction 225)
            ICE_BREAK -> (junction 225) [order 1] : [before(600,tick)&&...
                | hasChangedTo(SI_b_DCUCinchHomeSwt,0)]
          state INITIAL
            en:
            SO_b_MotorA=1;
            SO_b_MotorB=0;
            SO_e_MotorMode=1;
            //MotorA=Release Side
          state CHECKING
            en:
            SO_b_MotorA=0;
            SO_b_MotorB=0;
            SO_e_MotorMode=0;
            SL_e_CheckCycle++;
          state RESET
            en:
            SO_b_MotorA=0;
            SO_b_MotorB=1;
            SO_e_MotorMode=2;
          (default) -> NORMAL.ELECTRIC_DOOR.MAIN_PROGRESS.RELEASE.INITIAL
          NORMAL.ELECTRIC_DOOR.MAIN_PROGRESS.RELEASE.INITIAL -> NORMAL.ELECTRIC_DOOR.MAIN_PROGRESS.RELEASE.CHECKING : [after(30,tick)]
          NORMAL.ELECTRIC_DOOR.MAIN_PROGRESS.RELEASE.CHECKING -> NORMAL.ELECTRIC_DOOR.MAIN_PROGRESS.RELEASE.INITIAL [order 2] : [after(5,tick)&&...
              | SI_b_DoorAjarSts!=1&&...
              | SL_e_CheckCycle<2]
          NORMAL.ELECTRIC_DOOR.MAIN_PROGRESS.RELEASE.CHECKING -> NORMAL.ELECTRIC_DOOR.MAIN_PROGRESS.RELEASE.STEP2_OPEN [order 1] : [after(5,tick)&&...
              | SI_b_DoorAjarSts==1]
          NORMAL.ELECTRIC_DOOR.MAIN_PROGRESS.RELEASE.CHECKING -> NORMAL.ELECTRIC_DOOR.MAIN_PROGRESS.RELEASE.RESET [order 3] : [after(5,tick)&&...
              | SI_b_DoorAjarSts!=1&&...
              | SL_e_CheckCycle>=2]
          (junction 225) -> NORMAL.ELECTRIC_DOOR.MAIN_PROGRESS.RELEASE.RESET
        state IDLE
          en:
          SO_b_MotorA=0;
          SO_b_MotorB=0;
          SO_e_MotorMode=0;
          SO_b_Error=0;
        (default) -> NORMAL.ELECTRIC_DOOR.MAIN_PROGRESS.IDLE
        NORMAL.ELECTRIC_DOOR.MAIN_PROGRESS.IDLE -> NORMAL.ELECTRIC_DOOR.MAIN_PROGRESS.RELEASE : [hasChangedTO(SI_b_TriggerRelease,1)]
        NORMAL.ELECTRIC_DOOR.MAIN_PROGRESS.RELEASE.RESET -> NORMAL.ELECTRIC_DOOR.MAIN_PROGRESS.IDLE : [after(30,tick)]
    state NON_ELECTRIC_DOOR
      state MAIN_PROGRESS [parallel]
        settings: executionOrder=1
        state RELEASE
          en:
          SL_e_CheckCycle=0;
          state INITIAL
            en:
            SO_b_MotorA=1;
            SO_b_MotorB=0;
            SO_e_MotorMode=1;
            //MotorA=Release Side
          state CHECKING
            en:
            SO_b_MotorA=0;
            SO_b_MotorB=0;
            SO_e_MotorMode=0;
            SL_e_CheckCycle++;
          state STEP2_OPEN
            state IDLE
              en:
              SO_b_MotorA=0;
              SO_b_MotorB=0;
              SO_e_MotorMode=0;
            state WAITING
            state LAST_CHECK
            (default) -> NORMAL.NON_ELECTRIC_DOOR.MAIN_PROGRESS.RELEASE.STEP2_OPEN.IDLE
            NORMAL.NON_ELECTRIC_DOOR.MAIN_PROGRESS.RELEASE.STEP2_OPEN.WAITING -> (junction 251) : [after(5,tick)]
            NORMAL.NON_ELECTRIC_DOOR.MAIN_PROGRESS.RELEASE.STEP2_OPEN.IDLE -> NORMAL.NON_ELECTRIC_DOOR.MAIN_PROGRESS.RELEASE.STEP2_OPEN.WAITING [order 1] : [SI_b_DoorOpenSts==1]
            (junction 251) -> (junction 250)
            NORMAL.NON_ELECTRIC_DOOR.MAIN_PROGRESS.RELEASE.STEP2_OPEN.IDLE -> (junction 250) [order 2] : [before(270,tick)&&...
                | hasChangedTo(SI_b_DoorOpenSts,1)]
            (junction 250) -> (junction 242)
            NORMAL.NON_ELECTRIC_DOOR.MAIN_PROGRESS.RELEASE.STEP2_OPEN.IDLE -> NORMAL.NON_ELECTRIC_DOOR.MAIN_PROGRESS.RELEASE.STEP2_OPEN.LAST_CHECK [order 3] : [after(300,tick)&&...
                | SI_b_DoorOpenSts==0]
            NORMAL.NON_ELECTRIC_DOOR.MAIN_PROGRESS.RELEASE.STEP2_OPEN.LAST_CHECK -> (junction 242)
          state RESET
            en:
            SO_b_MotorA=0;
            SO_b_MotorB=1;
            SO_e_MotorMode=2;
          (default) -> NORMAL.NON_ELECTRIC_DOOR.MAIN_PROGRESS.RELEASE.INITIAL
          NORMAL.NON_ELECTRIC_DOOR.MAIN_PROGRESS.RELEASE.INITIAL -> NORMAL.NON_ELECTRIC_DOOR.MAIN_PROGRESS.RELEASE.CHECKING : [after(30,tick)]
          NORMAL.NON_ELECTRIC_DOOR.MAIN_PROGRESS.RELEASE.CHECKING -> NORMAL.NON_ELECTRIC_DOOR.MAIN_PROGRESS.RELEASE.STEP2_OPEN [order 1] : [after(5,tick)&&...
              | SI_b_DoorAjarSts==1]
          NORMAL.NON_ELECTRIC_DOOR.MAIN_PROGRESS.RELEASE.CHECKING -> NORMAL.NON_ELECTRIC_DOOR.MAIN_PROGRESS.RELEASE.INITIAL [order 2] : [after(5,tick)&&...
              | SI_b_DoorAjarSts!=1&&...
              | SL_e_CheckCycle<2]
          NORMAL.NON_ELECTRIC_DOOR.MAIN_PROGRESS.RELEASE.CHECKING -> NORMAL.NON_ELECTRIC_DOOR.MAIN_PROGRESS.RELEASE.RESET [order 3] : [after(5,tick)&&...
              | SI_b_DoorAjarSts!=1&&...
              | SL_e_CheckCycle>=2]
          (junction 242) -> NORMAL.NON_ELECTRIC_DOOR.MAIN_PROGRESS.RELEASE.RESET
        state IDLE
          en:
          SO_b_MotorA=0;
          SO_b_MotorB=0;
          SO_e_MotorMode=0;
        (default) -> NORMAL.NON_ELECTRIC_DOOR.MAIN_PROGRESS.IDLE
        NORMAL.NON_ELECTRIC_DOOR.MAIN_PROGRESS.IDLE -> NORMAL.NON_ELECTRIC_DOOR.MAIN_PROGRESS.RELEASE : [hasChangedTO(SI_b_TriggerRelease,1)]
        NORMAL.NON_ELECTRIC_DOOR.MAIN_PROGRESS.RELEASE.RESET -> NORMAL.NON_ELECTRIC_DOOR.MAIN_PROGRESS.IDLE : [after(30,tick)]
    (default) -> ELECTRIC_DOOR [order 1] : [SI_b_ElectricDoorCfg]
    (default) -> NON_ELECTRIC_DOOR [order 2]
  (default) -> STARTUP_SETTING
  STARTUP_SETTING -> NORMAL : [after(30,tick)]
  data: SO_b_MotorA output boolean; SI_b_TriggerRelease input boolean; SI_b_DoorOpenSts input boolean; SO_b_MotorB output boolean; SO_e_MotorMode output uint8; SI_b_DCUCinchHomeSwt input boolean; SO_b_Error output boolean; SI_b_ElectricDoorCfg input boolean; SI_b_DoorAjarSts input boolean
